simulink model "model_system_level_cycle"  (R2023a)
settings: Solver=VariableStepAuto  StartTime=0.0  StopTime=600  RelTol=1e-3  AbsTol=1e-3
libraries: fl_lib x9, nesl_utility x5, SimscapeFluids_lib x3
settings Model: Creator=ytang  LastModifiedBy=ytang
settings SolverCC: AutoScaleAbsTol=off  AlgebraicLoopSolver=TrustRegion  MaxZcPerStep=1
settings DebuggingCC: UnconnectedInputMsg=warning  UnconnectedOutputMsg=warning  UnconnectedLineMsg=warning  SymbolicDimsDataTypeCodeGenerationDiagnostic=none
settings ModelReferenceCC: EnableRefExpFcnMdlSchedulingChecks=on
settings SFSimCC: CustomCodeUndefinedFunction=UseInterfaceOnly
settings RTWCC: DLArmComputeVersion=19.05
settings SimscapeCC: SimscapeLogType=all  SimscapeLogSimulationStatistics=on  SimscapeLogDataHistory=10000

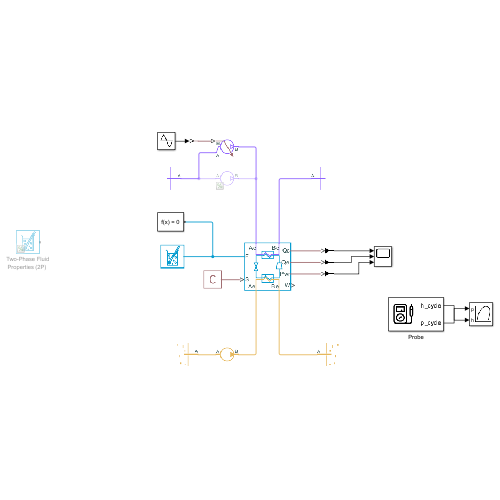
[thumbnail: Simulink's stored preview of the top-level diagram]
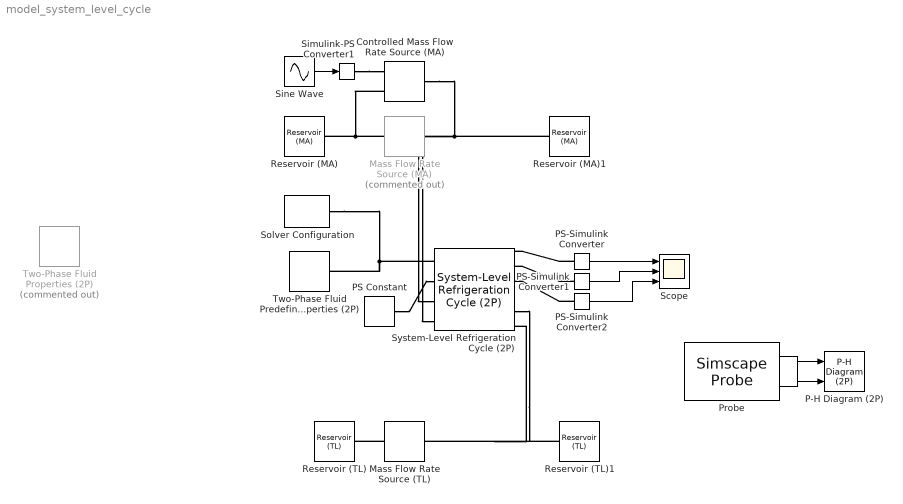
== system model_system_level_cycle ==
  Controlled Mass Flow Rate Source (MA) : fl_lib/Moist Air/Sources/Controlled Mass Flow Rate Source (MA)  power_spec=foundation.enum.power_spec.isentropic  area_A=1 m^2  area_B=1 m^2
      settings: InternalSimscapePortConfiguration="{\"Bottom\":[],\"Left\":[{\"id\":\"A\",\"label\":\"A\",\"type\":\"foundation.moist_air.moist_air\"},{\"id\":\"M\",\"label\":\"M\",\"type\":\"input\"}],\"Right\":[{\"id\":\"B\",\"label\":\"B\",\"type\":\"foundation.moist_air.moist_air\"}],\"Top\":[]}"
  Mass Flow Rate Source (MA) : fl_lib/Moist Air/Sources/Mass Flow Rate Source (MA)  Commented=on  power_spec=foundation.enum.power_spec.isentropic  mass_flow=1 kg/s  area_A=1 m^2  area_B=1 m^2
      settings: InternalSimscapePortConfiguration="{\"Bottom\":[],\"Left\":[{\"id\":\"A\",\"label\":\"A\",\"type\":\"foundation.moist_air.moist_air\"}],\"Right\":[{\"id\":\"B\",\"label\":\"B\",\"type\":\"foundation.moist_air.moist_air\"}],\"Top\":[]}"
  Mass Flow Rate Source (TL) : fl_lib/Thermal Liquid/Sources/Mass Flow Rate Source (TL)  power_spec=foundation.enum.power_spec.isentropic  commanded_mass_flow=0.2 kg/s  area=0.001 m^2
      settings: InternalSimscapePortConfiguration="{\"Bottom\":[],\"Left\":[{\"id\":\"A\",\"label\":\"A\",\"type\":\"foundation.thermal_liquid.thermal_liquid\"}],\"Right\":[{\"id\":\"B\",\"label\":\"B\",\"type\":\"foundation.thermal_liquid.thermal_liquid\"}],\"Top\":[]}"
  P-H Diagram (2P) : SimscapeFluids_lib/Two-Phase Fluid/Utilities/P-H Diagram (2P)
  PS Constant : fl_lib/Physical Signals/Sources/PS Constant  constant=1
  PS-Simulink Converter : nesl_utility/PS-Simulink Converter  PhysicalDomain=network_engine_domain  SubClassName=ps_output  LeftPortType=input  RightPortType=output  PseudoPeriodic=off  Frequencies=[]  VectorFormat=inherit  Unit=inherit  AffineConversion=off
  PS-Simulink Converter1 : nesl_utility/PS-Simulink Converter  PhysicalDomain=network_engine_domain  SubClassName=ps_output  LeftPortType=input  RightPortType=output  PseudoPeriodic=off  Frequencies=[]  VectorFormat=inherit  Unit=inherit  AffineConversion=off
  PS-Simulink Converter2 : nesl_utility/PS-Simulink Converter  PhysicalDomain=network_engine_domain  SubClassName=ps_output  LeftPortType=input  RightPortType=output  PseudoPeriodic=off  Frequencies=[]  VectorFormat=inherit  Unit=inherit  AffineConversion=off
  Probe : SimscapeProbe  BoundBlock=11  Variables={h_cycle, p_cycle}
  Reservoir (MA) : fl_lib/Moist Air/Elements/Reservoir (MA)  pressure_spec=foundation.enum.pressure_spec.atmospheric  reservoir_pressure=0.101325 MPa  temperature_spec=foundation.enum.temperature_spec.specified  reservoir_temperature=35 degC  moisture_spec=foundation.enum.moistureSpec.RelativeHumidity  reservoir_RH=0.5  reservoir_x_w=0.01  reservoir_y_w=0.01  reservoir_HR=0.01  reservoir_Tw=287 K  trace_gas_spec=foundation.enum.trace_gas_spec.mass_fraction  reservoir_x_g=0  reservoir_y_g=0.001  RH_ws=1  area_A=1 m^2
  Reservoir (MA)1 : fl_lib/Moist Air/Elements/Reservoir (MA)  pressure_spec=foundation.enum.pressure_spec.atmospheric  reservoir_pressure=0.101325 MPa  temperature_spec=foundation.enum.temperature_spec.specified  reservoir_temperature=35 degC  moisture_spec=foundation.enum.moistureSpec.RelativeHumidity  reservoir_RH=0.5  reservoir_x_w=0.01  reservoir_y_w=0.01  reservoir_HR=0.01  reservoir_Tw=287 K  trace_gas_spec=foundation.enum.trace_gas_spec.mass_fraction  reservoir_x_g=0  reservoir_y_g=0.001  RH_ws=1  area_A=1 m^2
  Reservoir (TL) : fl_lib/Thermal Liquid/Elements/Reservoir (TL)  pressure_spec=foundation.enum.pressure_spec.atmospheric  reservoir_pressure=0.101325 MPa  reservoir_temperature=20 degC  area=0.001 m^2
  Reservoir (TL)1 : fl_lib/Thermal Liquid/Elements/Reservoir (TL)  pressure_spec=foundation.enum.pressure_spec.atmospheric  reservoir_pressure=0.101325 MPa  reservoir_temperature=20 degC  area=0.001 m^2
  Scope : Scope  NumInputPorts=3
  Simulink-PS Converter1 : nesl_utility/Simulink-PS Converter  PhysicalDomain=network_engine_domain  SubClassName=ps_input  LeftPortType=input  RightPortType=output  PseudoPeriodic=off  Frequencies=[]  NoiseDistribution=none  NoiseParameters=[]  Unit=kg/s  AffineConversion=off  FilteringAndDerivatives=provide  SimscapeFilterOrder=1  InputFilterTimeConstant=0.001  UdotUserProvided=0
  Sine Wave : Sin  Amplitude=0.2  Bias=1  Frequency=2*pi/60  SampleTime=0
  Solver Configuration : nesl_utility/Solver Configuration  PhysicalDomain=network_engine_domain  SubClassName=solver  LeftPortType=input  RightPortType=generic  Tones=[]  Harmonics=[]  SimulateNoise=off  Profile=off  UseLocalSampling=off  EnableSwitchedLinearOptims=on  FrequencyDomain=off  UseCCode=off  RelTol=0.001  AbsTol=0.001  MinStep=1e-09  ToWorkspace=off  RevertToSquareIcSolve=off  NumHomotopyIterations=100  PhasorMode=off  PhasorModeNumHarmonics=1  ConsistencySolver=NEWTON_XTOL_AFTER_FTOL  IndexReductionMethod=None  DoDC=off  ResidualTolerance=1e-09  ConsistencyTolSource=GLOBAL  ConsistencyAbsTol=0.001  ConsistencyRelTol=0.001  ConsistencyTolFactor=0.001  UseLocalSolver=off  LocalSolverChoice=NE_BACKWARD_EULER_ADVANCER  ResolveIndetEquations=on  FunctionEvalNumThread=1  LocalSolverSampleTime=0.001  DoFixedCost=off  MaxNonlinIter=3  MaxModeIter=2  ComputeImpulses=off  ImpulseIterations=2  LinearAlgebra=auto  LinearAlgebraNumThread=0  EquationFormulation=NE_TIME_EF  DelaysMemoryBudget=1024  AutomaticFiltering=on  FilteringTimeConstant=0.001  PartitionStorageMethod=AS_NEEDED  PartitionMemoryBudget=1024  PartitionMethod=ROBUST
  System-Level Refrigeration Cycle (2P) : SimscapeFluids_lib/Two-Phase Fluid/Thermodynamic Cycles/System-Level Refrigeration Cycle (2P)  capacity_spec=fluids.two_phase_fluid.thermodynamic_cycles.enum.RefrigerationCycleCapacitySpec.CoolingLoad  Q_cond_nominal=15 kW  Q_evap_nominal=10 kW  mdot_nominal=0.005 kg/s  pressure_spec=fluids.two_phase_fluid.thermodynamic_cycles.enum.RefrigerationCyclePressureSpec.Pressure  p_cond_nominal=1.25 MPa  p_evap_nominal=0.3 MPa  T_cond_nominal=333.15 K  T_evap_nominal=273.15 K  delta_T_sub_nominal=5 deltaK  delta_T_sup_nominal=10 deltaK  delta_T_sup_static=5 deltaK  performance_spec=fluids.two_phase_fluid.thermodynamic_cycles.enum.RefrigerationCyclePerformanceSpec.CompressorEfficiency  COP_nominal=3  comp_eta_s=0.8  comp_eta_v_nominal=0.95  comp_eta_m=0.95  valve_max_fraction=5  valve_leak_fraction=1e-6  valve_smoothing_factor=0.01  volume_cond=0.001 m^3  volume_evap=0.001 m^3  receiver_volume=0.005 m^3  receiver_L_init=0.1  nominal_init=true  p_cond_init=1 MPa  p_evap_init=0.1 MPa  h_cond_init=[450, 250] kJ/kg  h_evap_init=[250, 400] kJ/kg  receiver_saturated_init=true  receiver_h_liq_init=500 kJ/kg  receiver_h_vap_init=3500 kJ/kg  cond_domain=fluids.two_phase_fluid.thermodynamic_cycles.enum.RefrigerationCycleFluidDomain.MoistAir  cond_mdot_nominal=1 kg/s  cond_delta_p_nominal=0.001 MPa  cond_pressure_spec=fluids.two_phase_fluid.thermodynamic_cycles.enum.RefrigerationCyclePressureSpec.Pressure  cond_p_in_nominal=0.101325 MPa  cond_T_sat_nominal=400 K  cond_inlet_spec=fluids.two_phase_fluid.thermodynamic_cycles.enum.RefrigerationCycleInletSpec.Enthalpy  cond_T_in_nominal=35 degC  cond_h_in_nominal=500 kJ/kg  cond_x_in_nominal=1  cond_inlet_moisture_spec=foundation.enum.moisture_spec.relative_humidity  cond_RH_in_nominal=0.5  cond_x_w_in_nominal=0.01  cond_y_w_in_nominal=0.01  cond_HR_in_nominal=0.01  cond_inlet_trace_gas_spec=foundation.enum.trace_gas_spec.mass_fraction  cond_x_g_in_nominal=0  cond_y_g_in_nominal=0.001  cond_volume=0.1 m^3  area_Ac=1 m^2  area_Bc=1 m^2  cond_wall_thermal_mass=false  cond_mass_wall=1 kg  cond_cp_wall=490 J/(K*kg)  cond_nominal_init=true  cond_p_init=0.101325 MPa  cond_energy_spec=foundation.enum.energy_spec.enthalpy  cond_T_init=293.15 K  cond_x_init=0.5  cond_alpha_init=0.5  cond_h_init=1500 kJ/kg  cond_u_init=1500 kJ/kg  cond_moisture_spec=foundation.enum.moisture_spec.relative_humidity  cond_RH_init=0.5  cond_x_w_init=0.01  cond_y_w_init=0.01  cond_HR_init=0.01  cond_trace_gas_spec=foundation.enum.trace_gas_spec.mass_fraction  cond_x_g_init=0.001  cond_y_g_init=0.001  cond_T_wall_init=293.15 K  cond_RH_ws=1  evap_domain=fluids.two_phase_fluid.thermodynamic_cycles.enum.RefrigerationCycleFluidDomain.ThermalLiquid  evap_mdot_nominal=0.2 kg/s  evap_delta_p_nominal=0.001 MPa  evap_pressure_spec=fluids.two_phase_fluid.thermodynamic_cycles.enum.RefrigerationCyclePressureSpec.Pressure  evap_p_in_nominal=0.101325 MPa  evap_T_sat_nominal=400 K  evap_inlet_spec=fluids.two_phase_fluid.thermodynamic_cycles.enum.RefrigerationCycleInletSpec.Enthalpy  evap_T_in_nominal=20 degC  evap_h_in_nominal=500 kJ/kg  evap_x_in_nominal=1  evap_inlet_moisture_spec=foundation.enum.moisture_spec.relative_humidity  evap_RH_in_nominal=0.1  evap_x_w_in_nominal=0.01  evap_y_w_in_nominal=0.01  evap_HR_in_nominal=0.01  evap_inlet_trace_gas_spec=foundation.enum.trace_gas_spec.mass_fraction  evap_x_g_in_nominal=0.001  evap_y_g_in_nominal=0.001  evap_volume=0.001 m^3  area_Ae=0.001 m^2  area_Be=0.001 m^2  evap_wall_thermal_mass=false  evap_mass_wall=1 kg  evap_cp_wall=490 J/(K*kg)  evap_nominal_init=true  evap_p_init=0.101325 MPa  evap_energy_spec=foundation.enum.energy_spec.enthalpy  evap_T_init=293.15 K  evap_x_init=0.5  evap_alpha_init=0.5  evap_h_init=1500 kJ/kg  evap_u_init=1500 kJ/kg  evap_moisture_spec=foundation.enum.moisture_spec.relative_humidity  evap_RH_init=0.5  evap_x_w_init=0.01  evap_y_w_init=0.01  evap_HR_init=0.01  evap_trace_gas_spec=foundation.enum.trace_gas_spec.mass_fraction  evap_x_g_init=0.001  evap_y_g_init=0.001  evap_T_wall_init=293.15 K  evap_RH_ws=1  cond_coeff_modify=false  cond_a_liq_refrig=0.023  cond_a_mix_refrig=0.005  cond_a_vap_refrig=0.023  cond_b_refrig=0.8  cond_c_refrig=0.33  cond_a_liq_extfld=0.023  cond_a_mix_extfld=0.005  cond_a_vap_extfld=0.023  cond_a_extfld=0.023  cond_b_extfld=0.8  cond_c_extfld=0.33  evap_coeff_modify=false  evap_a_liq_refrig=0.023  evap_a_mix_refrig=0.005  evap_a_vap_refrig=0.023  evap_b_refrig=0.8  evap_c_refrig=0.33  evap_a_liq_extfld=0.023  evap_a_mix_extfld=0.005  evap_a_vap_extfld=0.023  evap_a_extfld=0.023  evap_b_extfld=0.8  evap_c_extfld=0.33
      settings: InternalSimscapePortConfiguration="{\"Bottom\":[{\"id\":\"Ae_TL\",\"label\":\"Ae\",\"type\":\"foundation.thermal_liquid.thermal_liquid\"},{\"id\":\"Be_TL\",\"label\":\"Be\",\"type\":\"foundation.thermal_liquid.thermal_liquid\"}],\"Left\":[{\"id\":\"F\",\"label\":\"F\",\"type\":\"foundation.two_phase_fluid.two_phase_fluid\"},{\"id\":\"S\",\"label\":\"S\",\"type\":\"input\"}],\"Right\":[{\"id\":\"Qc\",\"label\":\"Qc\",\"type\":\"output\"},{\"id\":\"Qe\",\"label\":\"Qe\",\"type\":\"output\"},{\"id\":\"Pwr\",\"label\":\"Pwr\",\"type\":\"output\"},{\"id\":\"W\",\"label\":\"W\",\"type\":\"output\"}],\"Top\":[{\"id\":\"Ac_MA\",\"label\":\"Ac\",\"type\":\"foundation.moist_air.moist_air\"},{\"id\":\"Bc_MA\",\"label\":\"Bc\",\"type\":\"foundation.moist_air.moist_air\"}]}"
  Two-Phase Fluid Predefined Properties (2P) : SimscapeFluids_lib/Two-Phase Fluid/Utilities/Two-Phase Fluid Predefined Properties (2P)  fluid=fluids.two_phase_fluid.utilities.enum.Fluid.R134a  p_atm=0.101325 MPa  properties_range_check=simscape.enum.assert.action.error  q_rev=0.01 Pa
  "Two-Phase Fluid Properties (2P) " : fl_lib/Two-Phase Fluid/Utilities/Two-Phase Fluid Properties (2P)  Commented=on  u_min=r134aTables.u_min kJ/kg  u_max=r134aTables.u_max kJ/kg  p_TLU=r134aTables.p MPa  p_crit=r134aTables.p_crit MPa  critical_region=foundation.enum.critical_region.clip  p_crit_fraction=0.12  p_atm=0.101325 MPa  properties_range_check=simscape.enum.assert.action.error  q_rev=0.01 Pa  unorm_liq=r134aTables.liquid.unorm  v_liq=r134aTables.liquid.v m^3/kg  s_liq=r134aTables.liquid.s kJ/(kg*K)  T_liq=r134aTables.liquid.T K  nu_liq=r134aTables.liquid.nu mm^2/s  k_liq=r134aTables.liquid.k W/(m*K)  Pr_liq=r134aTables.liquid.Pr  u_sat_liq=r134aTables.liquid.u_sat kJ/kg  unorm_vap=r134aTables.vapor.unorm  v_vap=r134aTables.vapor.v m^3/kg  s_vap=r134aTables.vapor.s kJ/(kg*K)  T_vap=r134aTables.vapor.T K  nu_vap=r134aTables.vapor.nu mm^2/s  k_vap=r134aTables.vapor.k W/(m*K)  Pr_vap=r134aTables.vapor.Pr  u_sat_vap=r134aTables.vapor.u_sat kJ/kg
      settings: InternalSimscapePortConfiguration="{\"Bottom\":[],\"Left\":[],\"Right\":[{\"id\":\"A\",\"label\":\"\",\"type\":\"foundation.two_phase_fluid.two_phase_fluid\"}],\"Top\":[]}"
  wires:
  Probe/2 -> P-H Diagram (2P)/1
  Probe/1 -> P-H Diagram (2P)/2
  PS-Simulink Converter/1 -> Scope/1
  PS-Simulink Converter1/1 -> Scope/2
  PS-Simulink Converter2/1 -> Scope/3
  Sine Wave/1 -> Simulink-PS Converter1/1
  connections:
  System-Level Refrigeration Cycle (2P)/LConn1 -- Solver Configuration/RConn1 -- Two-Phase Fluid Predefined Properties (2P)/RConn1
  PS Constant/RConn1 -- System-Level Refrigeration Cycle (2P)/LConn2
  Controlled Mass Flow Rate Source (MA)/LConn1 -- Reservoir (MA)/LConn1 -- Mass Flow Rate Source (MA)/LConn1
  Reservoir (MA)1/LConn1 -- System-Level Refrigeration Cycle (2P)/LConn4
  Controlled Mass Flow Rate Source (MA)/RConn1 -- Mass Flow Rate Source (MA)/RConn1 -- System-Level Refrigeration Cycle (2P)/LConn3
  Reservoir (TL)1/LConn1 -- System-Level Refrigeration Cycle (2P)/RConn6
  System-Level Refrigeration Cycle (2P)/RConn5 -- Mass Flow Rate Source (TL)/RConn1
  Mass Flow Rate Source (TL)/LConn1 -- Reservoir (TL)/LConn1
  PS-Simulink Converter/LConn1 -- System-Level Refrigeration Cycle (2P)/RConn1
  PS-Simulink Converter1/LConn1 -- System-Level Refrigeration Cycle (2P)/RConn2
  PS-Simulink Converter2/LConn1 -- System-Level Refrigeration Cycle (2P)/RConn3
  Simulink-PS Converter1/RConn1 -- Controlled Mass Flow Rate Source (MA)/LConn2
